simulink model "sampleModel7424"  (R2017a)
settings: Solver=VariableStepAuto  StartTime=0.0  StopTime=10.0  RelTol=1e-3
undefined symbols (not defined in the file): DiscIntNeverNeededParam
libraries: simulink x211
(part 1 of 4)
settings Model: Creator=cyfuzz  LastModifiedBy=cyfuzz

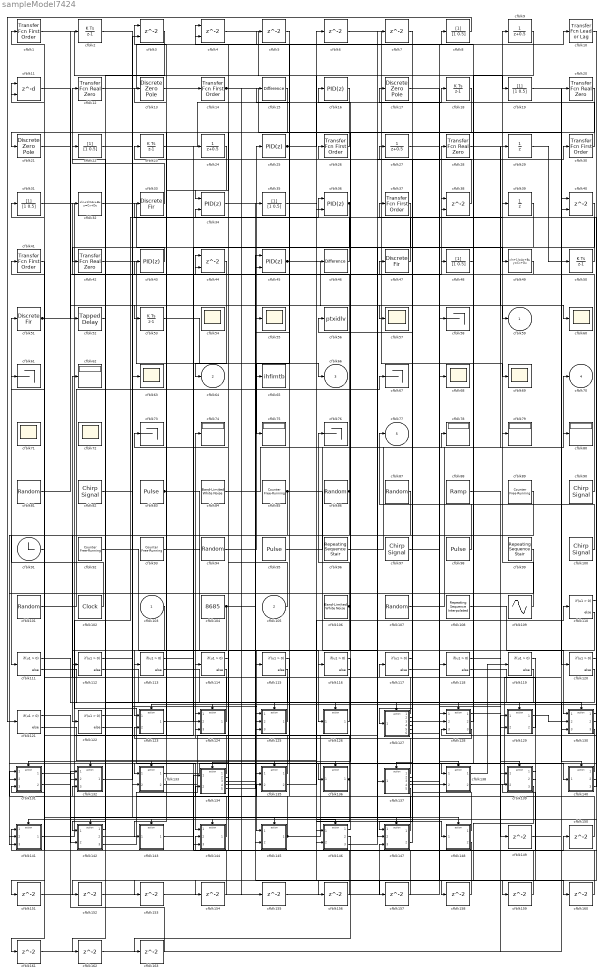
== system sampleModel7424 ==
  cfblk103 : Inport
  cfblk105 : Inport  Port=2
  cfblk{1,14,26,30,37,41} (6 alike) : simulink/Discrete/Transfer Fcn First Order  PoleZ=0.95  ICPrevOutput=0.0  DoSatur=off
      settings: SourceProductName=Simulink
  cfblk10 : simulink/Discrete/Transfer Fcn Lead or Lag  PoleZ=0.95  ZeroZ=0.75  ICPrevOutput=0.0  ICPrevInput=0.0  DoSatur=off
      settings: SourceProductName=Simulink  SourceProductBaseCode=SL
  cfblk{82,90,97,100} (4 alike) : simulink/Sources/Chirp Signal  f1=0.1  T=100  f2=1
  cfblk101 : UniformRandomNumber  SampleTime=0.1
  cfblk102 : DigitalClock
  cfblk104 : Constant  Value=8685
  cfblk106 : simulink/Sources/Band-Limited White Noise  Cov=[0.1]  Ts=0.1  seed=[23341]
  cfblk107 : RandomNumber  SampleTime=0.1
  cfblk108 : simulink/Sources/Repeating Sequence Interpolated  OutValues=[3 1 4 2 1].'  TimeValues=[0 0.1 0.5 0.6 1].'  LookUpMeth=Interpolation-Use End Values  tsamp=0.01  OutMin=[]  OutMax=[]  OutDataTypeStr=double  OutputDataTypeScalingMode=double  OutDataType=fixdt(0,8)  OutScaling=2^-10
  cfblk109 : Sin  SampleTime=0
  cfblk11 : Delay  DelayLengthSource=Input port  SampleTime=1
      settings: InputPortMap=u0,p1
  cfblk{110..122} (13 alike) : If  SampleTime=1
  cfblk{12,20,28,42} (4 alike) : simulink/Discrete/Transfer Fcn Real Zero  ZeroZ=0.75  ICPrevInput=0.0  DoSatur=off
      settings: SourceProductName=Simulink  SourceProductBaseCode=SL
  cfblk123 : Subsystem  TreatAsAtomicUnit=on
  cfblk124 : Subsystem  TreatAsAtomicUnit=on
  cfblk125 : Subsystem  TreatAsAtomicUnit=on
  cfblk126 : Subsystem  TreatAsAtomicUnit=on
  cfblk127 : Subsystem  TreatAsAtomicUnit=on
  cfblk128 : Subsystem  TreatAsAtomicUnit=on
  cfblk129 : Subsystem  TreatAsAtomicUnit=on
  cfblk13 : DiscreteZeroPole  Poles=[0 0.5]  Gain=1
  cfblk130 : Subsystem  TreatAsAtomicUnit=on
  cfblk131 : Subsystem  TreatAsAtomicUnit=on
  cfblk132 : Subsystem  TreatAsAtomicUnit=on
  cfblk133 : Subsystem  TreatAsAtomicUnit=on
  cfblk134 : Subsystem  TreatAsAtomicUnit=on
  cfblk135 : Subsystem  TreatAsAtomicUnit=on
  cfblk136 : Subsystem  TreatAsAtomicUnit=on
  cfblk137 : Subsystem  TreatAsAtomicUnit=on
  cfblk138 : Subsystem  TreatAsAtomicUnit=on
  cfblk139 : Subsystem  TreatAsAtomicUnit=on
  cfblk140 : Subsystem  TreatAsAtomicUnit=on
  cfblk141 : Subsystem  TreatAsAtomicUnit=on
  cfblk142 : Subsystem  TreatAsAtomicUnit=on
  cfblk143 : Subsystem  TreatAsAtomicUnit=on
  cfblk144 : Subsystem  TreatAsAtomicUnit=on
  cfblk145 : Subsystem  TreatAsAtomicUnit=on
  cfblk146 : Subsystem  TreatAsAtomicUnit=on
  cfblk147 : Subsystem  TreatAsAtomicUnit=on
  cfblk148 : Subsystem  TreatAsAtomicUnit=on
  cfblk{5..7,149..163} (18 alike) : Delay  SampleTime=1
  cfblk15 : simulink/Discrete/Difference  ICPrevInput=0.0  OutMin=[]  OutMax=[]  OutDataTypeStr=Inherit: Inherit via back propagation  OutDataType=fixdt(1, 16)  OutScaling=2^-10  DoSatur=off
  cfblk16 : simulink/Continuous/PID Controller  Controller=PID  TimeDomain=Discrete-time  SampleTime=1  IntegratorMethod=Forward Euler  FilterMethod=Forward Euler  Form=Parallel  UseFilter=on  ControllerParametersSource=internal  P=1  I=1  D=0  N=100  InitialConditionSource=internal  InitialConditionForIntegrator=0  InitialConditionForFilter=0  ExternalReset=none  LimitOutput=off  UpperSaturationLimit=inf  LowerSaturationLimit=-inf  LinearizeAsGain=off  AntiWindupMode=none  Kb=1  TrackingMode=off  Kt=1  PParamMin=[]  PParamMax=[]  IParamMin=[]  IParamMax=[]  DParamMin=[]  DParamMax=[]  NParamMin=[]  NParamMax=[]  KbParamMin=[]  KbParamMax=[]  KtParamMin=[]  KtParamMax=[]  POutMin=[]  POutMax=[]  IOutMin=[]  IOutMax=[]  DOutMin=[]  DOutMax=[]  NOutMin=[]  NOutMax=[]  KbOutMin=[]  KbOutMax=[]  KtOutMin=[]  KtOutMax=[]  IntegratorOutMin=[]  IntegratorOutMax=[]  FilterOutMin=[]  FilterOutMax=[]  SumOutMin=[]  SumOutMax=[]  SumI1OutMin=[]  SumI1OutMax=[]  SumI2OutMin=[]  SumI2OutMax=[]  SumI3OutMin=[]  SumI3OutMax=[]  SumDOutMin=[]  SumDOutMax=[]  SaturationOutMin=[]  SaturationOutMax=[]  IntegratorContinuousStateAttributes=''  IntegratorStateMustResolveToSignalObject=off  IntegratorRTWStateStorageClass=Auto  FilterContinuousStateAttributes=''  FilterStateMustResolveToSignalObject=off  FilterRTWStateStorageClass=Auto  DifferentiatorICPrevScaledInput=0  DifferentiatorOutMin=[]  DifferentiatorOutMax=[]  InitialConditionSetting=State (most efficient)
  cfblk17 : DiscreteZeroPole  Poles=[0 0.5]  Gain=1
  cfblk{2,18,23,50,53} (5 alike) : DiscreteIntegrator  InitialConditionSetting=State (most efficient)  ICPrevOutput=DiscIntNeverNeededParam  ICPrevScaledInput=DiscIntNeverNeededParam
  cfblk{8,19,22,31,35,48} (6 alike) : DiscreteFilter  SampleTime=1
  cfblk21 : DiscreteZeroPole  Poles=[0 0.5]  Gain=1
  cfblk24 : DiscreteTransferFcn  SampleTime=1
  cfblk25 : simulink/Continuous/PID Controller  Controller=PID  TimeDomain=Discrete-time  SampleTime=1  IntegratorMethod=Forward Euler  FilterMethod=Forward Euler  Form=Parallel  UseFilter=on  ControllerParametersSource=internal  P=1  I=1  D=0  N=100  InitialConditionSource=internal  InitialConditionForIntegrator=0  InitialConditionForFilter=0  ExternalReset=none  LimitOutput=off  UpperSaturationLimit=inf  LowerSaturationLimit=-inf  LinearizeAsGain=off  AntiWindupMode=none  Kb=1  TrackingMode=off  Kt=1  PParamMin=[]  PParamMax=[]  IParamMin=[]  IParamMax=[]  DParamMin=[]  DParamMax=[]  NParamMin=[]  NParamMax=[]  KbParamMin=[]  KbParamMax=[]  KtParamMin=[]  KtParamMax=[]  POutMin=[]  POutMax=[]  IOutMin=[]  IOutMax=[]  DOutMin=[]  DOutMax=[]  NOutMin=[]  NOutMax=[]  KbOutMin=[]  KbOutMax=[]  KtOutMin=[]  KtOutMax=[]  IntegratorOutMin=[]  IntegratorOutMax=[]  FilterOutMin=[]  FilterOutMax=[]  SumOutMin=[]  SumOutMax=[]  SumI1OutMin=[]  SumI1OutMax=[]  SumI2OutMin=[]  SumI2OutMax=[]  SumI3OutMin=[]  SumI3OutMax=[]  SumDOutMin=[]  SumDOutMax=[]  SaturationOutMin=[]  SaturationOutMax=[]  IntegratorContinuousStateAttributes=''  IntegratorStateMustResolveToSignalObject=off  IntegratorRTWStateStorageClass=Auto  FilterContinuousStateAttributes=''  FilterStateMustResolveToSignalObject=off  FilterRTWStateStorageClass=Auto  DifferentiatorICPrevScaledInput=0  DifferentiatorOutMin=[]  DifferentiatorOutMax=[]  InitialConditionSetting=State (most efficient)
  cfblk27 : DiscreteTransferFcn  SampleTime=1
  cfblk29 : UnitDelay
  cfblk{3..4,38,40,44} (5 alike) : Delay  ShowEnablePort=on  SampleTime=1
      settings: InputPortMap=u0,e6
  cfblk32 : DiscreteStateSpace
  cfblk33 : DiscreteFir  SampleTime=1
  cfblk34 : simulink/Continuous/PID Controller (2DOF)  Controller=PID  TimeDomain=Discrete-time  SampleTime=1  IntegratorMethod=Forward Euler  FilterMethod=Forward Euler  Form=Parallel  UseFilter=on  ControllerParametersSource=internal  P=1  I=1  D=0  N=100  b=1  c=1  InitialConditionSource=internal  InitialConditionForIntegrator=0  InitialConditionForFilter=0  ExternalReset=none  LimitOutput=off  UpperSaturationLimit=inf  LowerSaturationLimit=-inf  LinearizeAsGain=off  AntiWindupMode=none  Kb=1  TrackingMode=off  Kt=1  PParamMin=[]  PParamMax=[]  IParamMin=[]  IParamMax=[]  DParamMin=[]  DParamMax=[]  NParamMin=[]  NParamMax=[]  bParamMin=[]  bParamMax=[]  cParamMin=[]  cParamMax=[]  KbParamMin=[]  KbParamMax=[]  KtParamMin=[]  KtParamMax=[]  POutMin=[]  POutMax=[]  IOutMin=[]  IOutMax=[]  DOutMin=[]  DOutMax=[]  NOutMin=[]  NOutMax=[]  bOutMin=[]  bOutMax=[]  cOutMin=[]  cOutMax=[]  KbOutMin=[]  KbOutMax=[]  KtOutMin=[]  KtOutMax=[]  IntegratorOutMin=[]  IntegratorOutMax=[]  FilterOutMin=[]  FilterOutMax=[]  SumOutMin=[]  SumOutMax=[]  Sum1OutMin=[]  Sum1OutMax=[]  Sum2OutMin=[]  Sum2OutMax=[]  Sum3OutMin=[]  Sum3OutMax=[]  SumI1OutMin=[]  SumI1OutMax=[]  SumI2OutMin=[]  SumI2OutMax=[]  SumI3OutMin=[]  SumI3OutMax=[]  SumDOutMin=[]  SumDOutMax=[]  SaturationOutMin=[]  SaturationOutMax=[]  IntegratorContinuousStateAttributes=''  IntegratorStateMustResolveToSignalObject=off  IntegratorRTWStateStorageClass=Auto  FilterContinuousStateAttributes=''  FilterStateMustResolveToSignalObject=off  FilterRTWStateStorageClass=Auto  DifferentiatorICPrevScaledInput=0  DifferentiatorOutMin=[]  DifferentiatorOutMax=[]  InitialConditionSetting=State (most efficient)
  cfblk36 : simulink/Continuous/PID Controller (2DOF)  Controller=PID  TimeDomain=Discrete-time  SampleTime=1  IntegratorMethod=Forward Euler  FilterMethod=Forward Euler  Form=Parallel  UseFilter=on  ControllerParametersSource=internal  P=1  I=1  D=0  N=100  b=1  c=1  InitialConditionSource=internal  InitialConditionForIntegrator=0  InitialConditionForFilter=0  ExternalReset=none  LimitOutput=off  UpperSaturationLimit=inf  LowerSaturationLimit=-inf  LinearizeAsGain=off  AntiWindupMode=none  Kb=1  TrackingMode=off  Kt=1  PParamMin=[]  PParamMax=[]  IParamMin=[]  IParamMax=[]  DParamMin=[]  DParamMax=[]  NParamMin=[]  NParamMax=[]  bParamMin=[]  bParamMax=[]  cParamMin=[]  cParamMax=[]  KbParamMin=[]  KbParamMax=[]  KtParamMin=[]  KtParamMax=[]  POutMin=[]  POutMax=[]  IOutMin=[]  IOutMax=[]  DOutMin=[]  DOutMax=[]  NOutMin=[]  NOutMax=[]  bOutMin=[]  bOutMax=[]  cOutMin=[]  cOutMax=[]  KbOutMin=[]  KbOutMax=[]  KtOutMin=[]  KtOutMax=[]  IntegratorOutMin=[]  IntegratorOutMax=[]  FilterOutMin=[]  FilterOutMax=[]  SumOutMin=[]  SumOutMax=[]  Sum1OutMin=[]  Sum1OutMax=[]  Sum2OutMin=[]  Sum2OutMax=[]  Sum3OutMin=[]  Sum3OutMax=[]  SumI1OutMin=[]  SumI1OutMax=[]  SumI2OutMin=[]  SumI2OutMax=[]  SumI3OutMin=[]  SumI3OutMax=[]  SumDOutMin=[]  SumDOutMax=[]  SaturationOutMin=[]  SaturationOutMax=[]  IntegratorContinuousStateAttributes=''  IntegratorStateMustResolveToSignalObject=off  IntegratorRTWStateStorageClass=Auto  FilterContinuousStateAttributes=''  FilterStateMustResolveToSignalObject=off  FilterRTWStateStorageClass=Auto  DifferentiatorICPrevScaledInput=0  DifferentiatorOutMin=[]  DifferentiatorOutMax=[]  InitialConditionSetting=State (most efficient)
  cfblk39 : UnitDelay
  cfblk43 : simulink/Continuous/PID Controller  Controller=PID  TimeDomain=Discrete-time  SampleTime=1  IntegratorMethod=Forward Euler  FilterMethod=Forward Euler  Form=Parallel  UseFilter=on  ControllerParametersSource=internal  P=1  I=1  D=0  N=100  InitialConditionSource=internal  InitialConditionForIntegrator=0  InitialConditionForFilter=0  ExternalReset=none  LimitOutput=off  UpperSaturationLimit=inf  LowerSaturationLimit=-inf  LinearizeAsGain=off  AntiWindupMode=none  Kb=1  TrackingMode=off  Kt=1  PParamMin=[]  PParamMax=[]  IParamMin=[]  IParamMax=[]  DParamMin=[]  DParamMax=[]  NParamMin=[]  NParamMax=[]  KbParamMin=[]  KbParamMax=[]  KtParamMin=[]  KtParamMax=[]  POutMin=[]  POutMax=[]  IOutMin=[]  IOutMax=[]  DOutMin=[]  DOutMax=[]  NOutMin=[]  NOutMax=[]  KbOutMin=[]  KbOutMax=[]  KtOutMin=[]  KtOutMax=[]  IntegratorOutMin=[]  IntegratorOutMax=[]  FilterOutMin=[]  FilterOutMax=[]  SumOutMin=[]  SumOutMax=[]  SumI1OutMin=[]  SumI1OutMax=[]  SumI2OutMin=[]  SumI2OutMax=[]  SumI3OutMin=[]  SumI3OutMax=[]  SumDOutMin=[]  SumDOutMax=[]  SaturationOutMin=[]  SaturationOutMax=[]  IntegratorContinuousStateAttributes=''  IntegratorStateMustResolveToSignalObject=off  IntegratorRTWStateStorageClass=Auto  FilterContinuousStateAttributes=''  FilterStateMustResolveToSignalObject=off  FilterRTWStateStorageClass=Auto  DifferentiatorICPrevScaledInput=0  DifferentiatorOutMin=[]  DifferentiatorOutMax=[]  InitialConditionSetting=State (most efficient)
  cfblk45 : simulink/Continuous/PID Controller (2DOF)  Controller=PID  TimeDomain=Discrete-time  SampleTime=1  IntegratorMethod=Forward Euler  FilterMethod=Forward Euler  Form=Parallel  UseFilter=on  ControllerParametersSource=internal  P=1  I=1  D=0  N=100  b=1  c=1  InitialConditionSource=internal  InitialConditionForIntegrator=0  InitialConditionForFilter=0  ExternalReset=none  LimitOutput=off  UpperSaturationLimit=inf  LowerSaturationLimit=-inf  LinearizeAsGain=off  AntiWindupMode=none  Kb=1  TrackingMode=off  Kt=1  PParamMin=[]  PParamMax=[]  IParamMin=[]  IParamMax=[]  DParamMin=[]  DParamMax=[]  NParamMin=[]  NParamMax=[]  bParamMin=[]  bParamMax=[]  cParamMin=[]  cParamMax=[]  KbParamMin=[]  KbParamMax=[]  KtParamMin=[]  KtParamMax=[]  POutMin=[]  POutMax=[]  IOutMin=[]  IOutMax=[]  DOutMin=[]  DOutMax=[]  NOutMin=[]  NOutMax=[]  bOutMin=[]  bOutMax=[]  cOutMin=[]  cOutMax=[]  KbOutMin=[]  KbOutMax=[]  KtOutMin=[]  KtOutMax=[]  IntegratorOutMin=[]  IntegratorOutMax=[]  FilterOutMin=[]  FilterOutMax=[]  SumOutMin=[]  SumOutMax=[]  Sum1OutMin=[]  Sum1OutMax=[]  Sum2OutMin=[]  Sum2OutMax=[]  Sum3OutMin=[]  Sum3OutMax=[]  SumI1OutMin=[]  SumI1OutMax=[]  SumI2OutMin=[]  SumI2OutMax=[]  SumI3OutMin=[]  SumI3OutMax=[]  SumDOutMin=[]  SumDOutMax=[]  SaturationOutMin=[]  SaturationOutMax=[]  IntegratorContinuousStateAttributes=''  IntegratorStateMustResolveToSignalObject=off  IntegratorRTWStateStorageClass=Auto  FilterContinuousStateAttributes=''  FilterStateMustResolveToSignalObject=off  FilterRTWStateStorageClass=Auto  DifferentiatorICPrevScaledInput=0  DifferentiatorOutMin=[]  DifferentiatorOutMax=[]  InitialConditionSetting=State (most efficient)
  cfblk46 : simulink/Discrete/Difference  ICPrevInput=0.0  OutMin=[]  OutMax=[]  OutDataTypeStr=Inherit: Inherit via back propagation  OutDataType=fixdt(1, 16)  OutScaling=2^-10  DoSatur=off
  cfblk47 : DiscreteFir  SampleTime=1
  cfblk49 : DiscreteStateSpace
  cfblk51 : DiscreteFir  SampleTime=1
  cfblk52 : simulink/Discrete/Tapped Delay  vinit=0.0  samptime=-1  NumDelays=1  DelayOrder=Oldest  includeCurrent=off
  cfblk{54..55,57,60,63,68..69,71..72} (9 alike) : Scope
      cfblk54 settings: Floating=on
      cfblk71 settings: Floating=on
      cfblk72 settings: Floating=on
  cfblk56 : ToWorkspace  VariableName=ptxidlv  SaveFormat=Timeseries  SampleTime=-1
  cfblk{58,61,67,73,76} (5 alike) : Terminator
  cfblk{62,74..75,78..80} (6 alike) : Display
  cfblk65 : ToWorkspace  VariableName=ihfimtb  SaveFormat=Timeseries  SampleTime=-1
  cfblk81 : RandomNumber  SampleTime=0.1
  cfblk83 : DiscretePulseGenerator  PulseType=Time based  Period=10  PulseWidth=5
  cfblk84 : simulink/Sources/Band-Limited White Noise  Cov=[0.1]  Ts=0.1  seed=[23341]
  cfblk{85,89,92..93} (4 alike) : simulink/Sources/Counter Free-Running  NumBits=16  tsamp=-1
  cfblk86 : UniformRandomNumber  SampleTime=0.1
  cfblk87 : RandomNumber  SampleTime=0.1
  cfblk88 : simulink/Sources/Ramp  slope=1  start=0  X0=0
  cfblk9 : DiscreteTransferFcn  SampleTime=1
  cfblk91 : Clock
  cfblk94 : UniformRandomNumber  SampleTime=0.1
  cfblk95 : DiscretePulseGenerator  PulseType=Time based  Period=10  PulseWidth=5
  cfblk96 : simulink/Sources/Repeating Sequence Stair  OutValues=[3 1 4 2 1].'  tsamp=-1  OutMin=[]  OutMax=[]  OutDataTypeStr=double  OutputDataTypeScalingMode=double  OutDataType=fixdt(0,8)  ConRadixGroup=Best Precision: Vector-wise  OutScaling=2^-12
  cfblk98 : DiscretePulseGenerator  PulseType=Time based  Period=10  PulseWidth=5
  cfblk99 : simulink/Sources/Repeating Sequence Stair  OutValues=[3 1 4 2 1].'  tsamp=-1  OutMin=[]  OutMax=[]  OutDataTypeStr=double  OutputDataTypeScalingMode=double  OutDataType=fixdt(0,8)  ConRadixGroup=Best Precision: Vector-wise  OutScaling=2^-12
  cfblk59 : Outport
  cfblk64 : Outport  Port=2
  cfblk66 : Outport  Port=3
  cfblk70 : Outport  Port=4
  cfblk77 : Outport  Port=5
  wires:
  cfblk29/1 -> cfblk50/1
  cfblk23/1 -> cfblk18/1
  cfblk48/1 -> cfblk4/1
  cfblk109/1 -> cfblk9/1
  cfblk93/1 -> cfblk126/1(cfblk1)
  cfblk100/1 -> cfblk77/1
  cfblk138/1(cfblk2) -> cfblk119/1
  cfblk105/1 -> cfblk73/1
  cfblk102/1 -> cfblk51/1
  cfblk141/1(cfblk2) -> cfblk36/1
  cfblk92/1 -> cfblk145/1(cfblk1)
  cfblk42/1 -> cfblk66/1
  cfblk50/1 -> cfblk16/1
  cfblk83/1 -> cfblk115/1, cfblk146/1(cfblk1)
  cfblk94/1 -> cfblk25/1
  cfblk87/1 -> cfblk111/1
  cfblk84/1 -> cfblk78/1
  cfblk8/1 -> cfblk121/1
  cfblk45/1 -> cfblk59/1, cfblk5/1
  cfblk126/1(cfblk2) -> cfblk23/1
  cfblk33/1 -> cfblk12/1
  cfblk12/1 -> cfblk8/1
  cfblk95/1 -> cfblk70/1
  cfblk6/1 -> cfblk69/1
  cfblk108/1 -> cfblk130/1(cfblk1)
  cfblk146/1(cfblk2) -> cfblk26/1
  cfblk25/1 -> cfblk6/1, cfblk148/1(cfblk1)
  cfblk132/1(cfblk2) -> cfblk63/1
  cfblk4/1 -> cfblk19/1
  cfblk20/1 -> cfblk116/1
  cfblk14/1 -> cfblk120/1, cfblk155/1
  cfblk96/1 -> cfblk29/1
  cfblk13/1 -> cfblk14/1
  cfblk10/1 -> cfblk141/1(cfblk1)
  cfblk15/1 -> cfblk133/1(cfblk1)
  cfblk17/1 -> cfblk58/1
  cfblk53/1 -> cfblk75/1
  cfblk89/1 -> cfblk122/1
  cfblk98/1 -> cfblk47/1
  cfblk7/1 -> cfblk127/1(cfblk1)
  cfblk31/1 -> cfblk144/1(cfblk1)
  cfblk136/1(cfblk2) -> cfblk1/1, cfblk146/2(cfblk10)
  cfblk47/1 -> cfblk37/1
  cfblk124/1(cfblk2) -> cfblk61/1
  cfblk138/2(cfblk7) -> cfblk20/1
  cfblk137/1(cfblk2) -> cfblk55/1
  cfblk134/1(cfblk2) -> cfblk43/1
  cfblk9/1 -> cfblk138/1(cfblk1)
  cfblk30/1 -> cfblk17/1
  cfblk133/1(cfblk2) -> cfblk140/1(cfblk1)
  cfblk123/1(cfblk2) -> cfblk74/1
  cfblk38/1 -> cfblk13/1
  cfblk101/1 -> cfblk7/1
  cfblk97/1 -> cfblk138/2(cfblk6)
  cfblk5/1 -> cfblk65/1
  cfblk46/1 -> cfblk3/1
  cfblk3/1 -> cfblk142/1(cfblk1)
  cfblk1/1 -> cfblk46/1
  cfblk44/1 -> cfblk64/1
  cfblk16/1 -> cfblk36/2
  cfblk91/1 -> cfblk31/1
  cfblk145/1(cfblk2) -> cfblk79/1, cfblk132/3(cfblk14)
  cfblk131/1(cfblk2) -> cfblk24/1
  cfblk81/1 -> cfblk2/1
  cfblk144/1(cfblk2) -> cfblk41/1
  cfblk86/1 -> cfblk32/1, cfblk141/3(cfblk14)
  cfblk21/1 -> cfblk52/1
  cfblk148/1(cfblk2) -> cfblk27/1
  cfblk51/1 -> cfblk11/1, cfblk48/1
  cfblk82/1 -> cfblk3/2
  cfblk137/2(cfblk11) -> cfblk35/1
  cfblk127/1(cfblk2) -> cfblk11/2
  cfblk90/1 -> cfblk28/1
  cfblk103/1 -> cfblk123/1(cfblk1)
  cfblk18/1 -> cfblk34/1
  cfblk2/1 -> cfblk57/1
  cfblk28/1 -> cfblk60/1
  cfblk127/2(cfblk13) -> cfblk123/2(cfblk10)
  cfblk106/1 -> cfblk76/1, cfblk125/2(cfblk9)
  cfblk129/1(cfblk2) -> cfblk130/2(cfblk7)
  cfblk43/1 -> cfblk42/1
  cfblk148/2(cfblk17) -> cfblk144/2(cfblk12)
  cfblk11/1 -> cfblk53/1
  cfblk135/1(cfblk2) -> cfblk124/1(cfblk1)
  cfblk134/2(cfblk14) -> cfblk34/2
  cfblk127/3(cfblk14) -> cfblk10/1
  cfblk134/3(cfblk15) -> cfblk45/1
  cfblk19/1 -> cfblk40/2
  cfblk142/1(cfblk2) -> cfblk22/1
  cfblk131/2(cfblk15) -> cfblk142/2(cfblk13)
  cfblk129/2(cfblk9) -> cfblk117/1
  cfblk107/1 -> cfblk80/1
  cfblk39/1 -> cfblk145/2(cfblk16)
  cfblk26/1 -> cfblk21/1
  cfblk32/1 -> cfblk49/1
  cfblk147/1(cfblk2) -> cfblk15/1
  cfblk128/2(cfblk11) -> cfblk38/1
  cfblk104/1 -> cfblk135/1(cfblk1), cfblk112/1
  cfblk27/1 -> cfblk129/2(cfblk8)
  cfblk36/1 -> cfblk124/2(cfblk12), cfblk125/3(cfblk10)
  cfblk85/1 -> cfblk137/1(cfblk1), cfblk143/1(cfblk1), cfblk133/2(cfblk16)
  cfblk40/1 -> cfblk147/1(cfblk1)
  cfblk134/4(cfblk16) -> cfblk67/1
  cfblk147/2(cfblk12) -> cfblk44/1
  cfblk142/2(cfblk14) -> cfblk39/1
  cfblk125/1(cfblk2) -> cfblk62/1
  cfblk99/1 -> cfblk141/2(cfblk13)
  cfblk49/1 -> cfblk44/2
  cfblk22/1 -> cfblk125/1(cfblk1)
  cfblk37/1 -> cfblk147/2(cfblk10)
  cfblk146/3(cfblk12) -> cfblk30/1
  cfblk133/2(cfblk17) -> cfblk38/2
  cfblk128/3(cfblk12) -> cfblk124/3(cfblk13)
  cfblk127/4(cfblk15) -> cfblk56/1
  cfblk127/5(cfblk16) -> cfblk136/1(cfblk1)
  cfblk88/1 -> cfblk139/1(cfblk1)
  cfblk142/3(cfblk15) -> cfblk135/2(cfblk13)
  cfblk140/1(cfblk2) -> cfblk131/2(cfblk13)
  cfblk140/2(cfblk7) -> cfblk132/2(cfblk13)
  cfblk130/1(cfblk2) -> cfblk128/3(cfblk10)
  cfblk140/3(cfblk8) -> cfblk33/1
  cfblk127/6(cfblk17) -> cfblk68/1
  cfblk135/2(cfblk14) -> cfblk110/1
  cfblk134/5(cfblk17) -> cfblk45/2
  cfblk24/1 -> cfblk113/1
  cfblk130/3(cfblk10) -> cfblk144/3(cfblk13)
  cfblk110/1 -> cfblk123/Action
  cfblk110/2 -> cfblk124/Action
  cfblk111/1 -> cfblk125/Action
  cfblk111/2 -> cfblk126/Action
  cfblk112/1 -> cfblk127/Action
  cfblk112/2 -> cfblk128/Action
  cfblk113/1 -> cfblk129/Action
  cfblk113/2 -> cfblk130/Action
  cfblk114/1 -> cfblk131/Action
  cfblk114/2 -> cfblk132/Action
  cfblk115/1 -> cfblk133/Action
  cfblk115/2 -> cfblk134/Action
  cfblk116/1 -> cfblk135/Action
  cfblk116/2 -> cfblk136/Action
  cfblk117/1 -> cfblk137/Action
  cfblk117/2 -> cfblk138/Action
  cfblk118/1 -> cfblk139/Action
  cfblk118/2 -> cfblk140/Action
  cfblk119/1 -> cfblk141/Action
  cfblk119/2 -> cfblk142/Action
  cfblk120/1 -> cfblk143/Action
  cfblk120/2 -> cfblk144/Action
  cfblk121/1 -> cfblk145/Action
  cfblk121/2 -> cfblk146/Action
  cfblk122/1 -> cfblk147/Action
  cfblk122/2 -> cfblk148/Action
  cfblk128/1(cfblk2) -> cfblk149/1
  cfblk149/1 -> cfblk40/1
  cfblk143/1(cfblk2) -> cfblk150/1
  cfblk150/1 -> cfblk131/1(cfblk1)
  cfblk41/1 -> cfblk151/1
  cfblk151/1 -> cfblk128/2(cfblk9)
  cfblk139/1(cfblk2) -> cfblk152/1
  cfblk152/1 -> cfblk128/1(cfblk1)
  cfblk139/2(cfblk9) -> cfblk153/1
  cfblk153/1 -> cfblk147/3(cfblk11)
  cfblk139/3(cfblk10) -> cfblk154/1
  cfblk154/1 -> cfblk131/3(cfblk14)
  cfblk155/1 -> cfblk118/1
  cfblk130/2(cfblk9) -> cfblk156/1
  cfblk156/1 -> cfblk134/2(cfblk13)
  cfblk34/1 -> cfblk157/1
  cfblk157/1 -> cfblk114/1
  cfblk35/1 -> cfblk158/1
  cfblk158/1 -> cfblk4/2
  cfblk137/3(cfblk12) -> cfblk159/1
  cfblk159/1 -> cfblk134/1(cfblk1)
  cfblk137/4(cfblk13) -> cfblk160/1
  cfblk160/1 -> cfblk139/2(cfblk8)
  cfblk137/5(cfblk14) -> cfblk161/1
  cfblk161/1 -> cfblk130/3(cfblk8)
  cfblk52/1 -> cfblk162/1
  cfblk162/1 -> cfblk129/1(cfblk1)
  cfblk146/2(cfblk11) -> cfblk163/1
  cfblk163/1 -> cfblk132/1(cfblk1)

== system sampleModel7424/cfblk123 ==
  cfblk1 : Inport
  cfblk10 : Inport  Port=2
  Action Port : ActionPort  ActionType=then
  cfblk3 : UnitDelay  SampleTime=-1
  cfblk4 : simulink/Continuous/PID Controller  Controller=PID  TimeDomain=Discrete-time  SampleTime=-1  IntegratorMethod=Forward Euler  FilterMethod=Forward Euler  Form=Parallel  UseFilter=on  ControllerParametersSource=internal  P=1  I=1  D=0  N=100  InitialConditionSource=internal  InitialConditionForIntegrator=0  InitialConditionForFilter=0  ExternalReset=none  LimitOutput=off  UpperSaturationLimit=inf  LowerSaturationLimit=-inf  LinearizeAsGain=off  AntiWindupMode=none  Kb=1  TrackingMode=off  Kt=1  PParamMin=[]  PParamMax=[]  IParamMin=[]  IParamMax=[]  DParamMin=[]  DParamMax=[]  NParamMin=[]  NParamMax=[]  KbParamMin=[]  KbParamMax=[]  KtParamMin=[]  KtParamMax=[]  POutMin=[]  POutMax=[]  IOutMin=[]  IOutMax=[]  DOutMin=[]  DOutMax=[]  NOutMin=[]  NOutMax=[]  KbOutMin=[]  KbOutMax=[]  KtOutMin=[]  KtOutMax=[]  IntegratorOutMin=[]  IntegratorOutMax=[]  FilterOutMin=[]  FilterOutMax=[]  SumOutMin=[]  SumOutMax=[]  SumI1OutMin=[]  SumI1OutMax=[]  SumI2OutMin=[]  SumI2OutMax=[]  SumI3OutMin=[]  SumI3OutMax=[]  SumDOutMin=[]  SumDOutMax=[]  SaturationOutMin=[]  SaturationOutMax=[]  IntegratorContinuousStateAttributes=''  IntegratorStateMustResolveToSignalObject=off  IntegratorRTWStateStorageClass=Auto  FilterContinuousStateAttributes=''  FilterStateMustResolveToSignalObject=off  FilterRTWStateStorageClass=Auto  DifferentiatorICPrevScaledInput=0  DifferentiatorOutMin=[]  DifferentiatorOutMax=[]  InitialConditionSetting=State (most efficient)
  cfblk5 : DiscreteTransferFcn
  cfblk6 : DiscreteIntegrator  InitialConditionSetting=State (most efficient)  SampleTime=-1  ICPrevOutput=DiscIntNeverNeededParam  ICPrevScaledInput=DiscIntNeverNeededParam
  cfblk7 : Delay
  cfblk8 : simulink/Discrete/Tapped Delay  vinit=0.0  samptime=-1  NumDelays=1  DelayOrder=Oldest  includeCurrent=off
  cfblk9 : DiscreteTransferFcn
  cfblk2 : Outport
  wires:
  cfblk4/1 -> cfblk8/1
  cfblk9/1 -> cfblk2/1
  cfblk6/1 -> cfblk7/1
  cfblk7/1 -> cfblk3/1
  cfblk10/1 -> cfblk4/1
  cfblk1/1 -> cfblk9/1
  cfblk3/1 -> cfblk5/1
  cfblk8/1 -> cfblk6/1

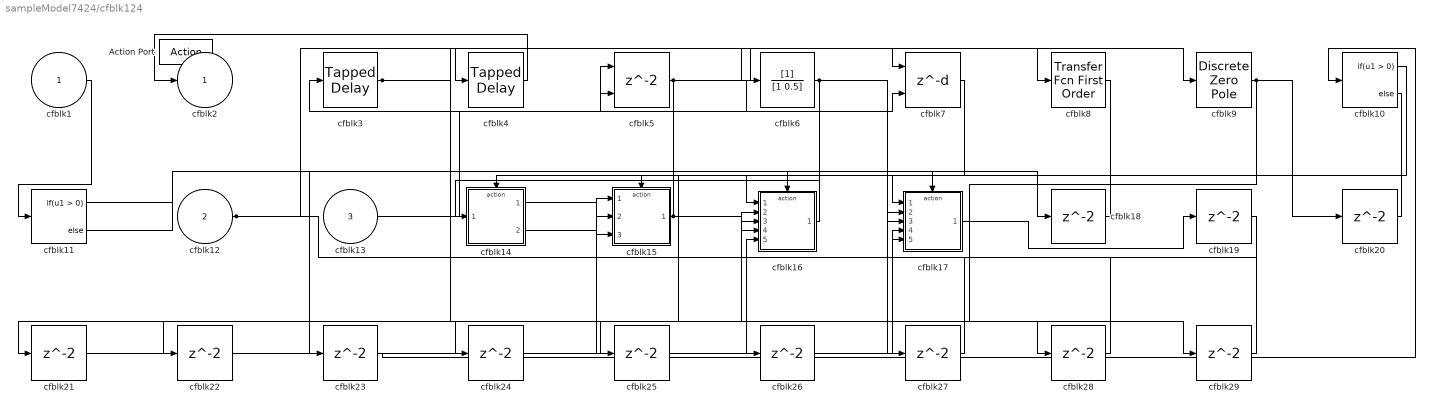
== system sampleModel7424/cfblk124 ==
  cfblk1 : Inport
  cfblk12 : Inport  Port=2
  cfblk13 : Inport  Port=3
  Action Port : ActionPort  ActionType=else
  cfblk10 : If  SampleTime=1
  cfblk11 : If  SampleTime=1
  cfblk14 : Subsystem  TreatAsAtomicUnit=on
  cfblk15 : Subsystem  TreatAsAtomicUnit=on
  cfblk16 : Subsystem  TreatAsAtomicUnit=on
  cfblk17 : Subsystem  TreatAsAtomicUnit=on
  cfblk{18..29} (12 alike) : Delay
  cfblk3 : simulink/Discrete/Tapped Delay  vinit=0.0  samptime=-1  NumDelays=1  DelayOrder=Oldest  includeCurrent=off
  cfblk4 : simulink/Discrete/Tapped Delay  vinit=0.0  samptime=-1  NumDelays=1  DelayOrder=Oldest  includeCurrent=off
  cfblk5 : Delay  ShowEnablePort=on
      settings: InputPortMap=u0,e6
  cfblk6 : DiscreteFilter
  cfblk7 : Delay  DelayLengthSource=Input port
      settings: InputPortMap=u0,p1
  cfblk8 : simulink/Discrete/Transfer Fcn First Order  PoleZ=0.95  ICPrevOutput=0.0  DoSatur=off
      settings: SourceProductName=Simulink
  cfblk9 : DiscreteZeroPole  Poles=[0 0.5]  Gain=1  SampleTime=-1
  cfblk2 : Outport
  wires:
  cfblk15/1(cfblk2) -> cfblk3/1, cfblk5/1, cfblk27/1
  cfblk1/1 -> cfblk11/1
  cfblk5/1 -> cfblk7/1, cfblk8/1, cfblk23/1
  cfblk12/1 -> cfblk4/1, cfblk17/4(cfblk14)
  cfblk13/1 -> cfblk7/2
  cfblk16/1(cfblk2) -> cfblk6/1
  cfblk3/1 -> cfblk9/1, cfblk5/2, cfblk18/1, cfblk25/1, cfblk26/1
  cfblk14/1(cfblk2) -> cfblk15/3(cfblk16)
  cfblk9/1 -> cfblk20/1, cfblk21/1
  cfblk6/1 -> cfblk14/1(cfblk1), cfblk29/1
  cfblk4/1 -> cfblk2/1
  cfblk10/1 -> cfblk14/Action
  cfblk10/2 -> cfblk15/Action
  cfblk11/1 -> cfblk16/Action
  cfblk11/2 -> cfblk17/Action
  cfblk18/1 -> cfblk17/1(cfblk1)
  cfblk17/1(cfblk2) -> cfblk19/1
  cfblk19/1 -> cfblk15/2(cfblk15)
  cfblk20/1 -> cfblk16/1(cfblk1)
  cfblk21/1 -> cfblk17/3(cfblk13)
  cfblk7/1 -> cfblk22/1
  cfblk22/1 -> cfblk17/2(cfblk12)
  cfblk23/1 -> cfblk10/1
  cfblk8/1 -> cfblk24/1
  cfblk24/1 -> cfblk15/1(cfblk1)
  cfblk25/1 -> cfblk16/5(cfblk14)
  cfblk26/1 -> cfblk17/5(cfblk15)
  cfblk27/1 -> cfblk16/3(cfblk12)
  cfblk14/2(cfblk7) -> cfblk28/1
  cfblk28/1 -> cfblk16/2(cfblk11)
  cfblk29/1 -> cfblk16/4(cfblk13)

== system sampleModel7424/cfblk125 ==
  cfblk1 : Inport
  cfblk9 : Inport  Port=2
  cfblk10 : Inport  Port=3
  Action Port : ActionPort  ActionType=then
  cfblk11 : Subsystem  TreatAsAtomicUnit=on
  cfblk12 : Subsystem  TreatAsAtomicUnit=on
  cfblk13 : Delay
  cfblk14 : Delay
  cfblk3 : simulink/Discrete/Transfer Fcn Real Zero  ZeroZ=0.75  ICPrevInput=0.0  DoSatur=off
      settings: SourceProductName=Simulink  SourceProductBaseCode=SL
  cfblk4 : Delay  DelayLengthSource=Input port
      settings: InputPortMap=u0,p1
  cfblk5 : simulink/Discrete/Transfer Fcn Lead or Lag  PoleZ=0.95  ZeroZ=0.75  ICPrevOutput=0.0  ICPrevInput=0.0  DoSatur=off
      settings: SourceProductName=Simulink  SourceProductBaseCode=SL
  cfblk6 : simulink/Discrete/Transfer Fcn Lead or Lag  PoleZ=0.95  ZeroZ=0.75  ICPrevOutput=0.0  ICPrevInput=0.0  DoSatur=off
      settings: SourceProductName=Simulink  SourceProductBaseCode=SL
  cfblk7 : DiscreteIntegrator  InitialConditionSetting=State (most efficient)  SampleTime=-1  ICPrevOutput=DiscIntNeverNeededParam  ICPrevScaledInput=DiscIntNeverNeededParam
  cfblk8 : If  SampleTime=1
  cfblk2 : Outport
  wires:
  cfblk4/1 -> cfblk5/1
  cfblk7/1 -> cfblk12/1(cfblk1)
  cfblk9/1 -> cfblk6/1
  cfblk10/1 -> cfblk2/1
  cfblk6/1 -> cfblk3/1
  cfblk11/2(cfblk13) -> cfblk4/2
  cfblk1/1 -> cfblk7/1
  cfblk3/1 -> cfblk11/1(cfblk1)
  cfblk12/1(cfblk2) -> cfblk11/2(cfblk12)
  cfblk8/1 -> cfblk11/Action
  cfblk8/2 -> cfblk12/Action
  cfblk11/1(cfblk2) -> cfblk13/1
  cfblk13/1 -> cfblk8/1
  cfblk5/1 -> cfblk14/1
  cfblk14/1 -> cfblk4/1

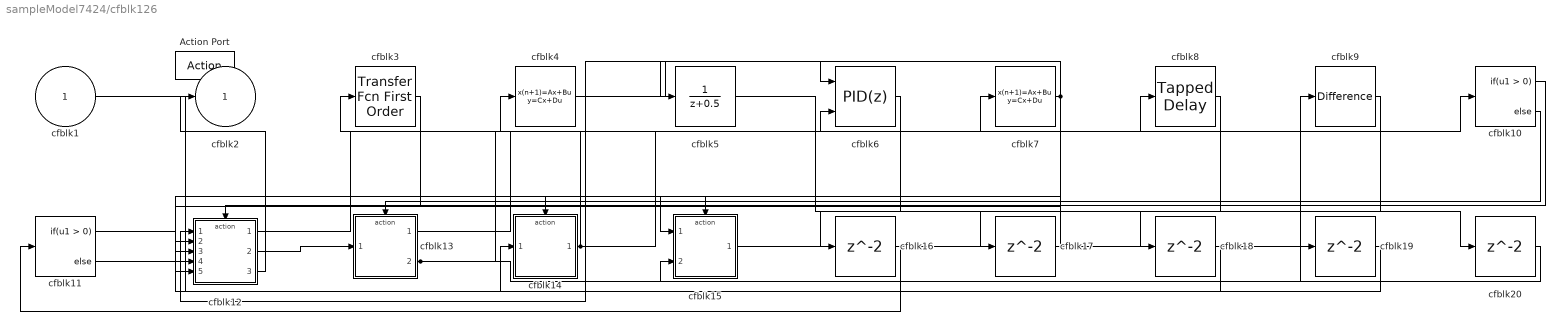
== system sampleModel7424/cfblk126 ==
  cfblk1 : Inport
  Action Port : ActionPort  ActionType=else
  cfblk10 : If  SampleTime=1
  cfblk11 : If  SampleTime=1
  cfblk12 : Subsystem  TreatAsAtomicUnit=on
  cfblk13 : Subsystem  TreatAsAtomicUnit=on
  cfblk14 : Subsystem  TreatAsAtomicUnit=on
  cfblk15 : Subsystem  TreatAsAtomicUnit=on
  cfblk{16..20} (5 alike) : Delay
  cfblk3 : simulink/Discrete/Transfer Fcn First Order  PoleZ=0.95  ICPrevOutput=0.0  DoSatur=off
      settings: SourceProductName=Simulink
  cfblk4 : DiscreteStateSpace  SampleTime=-1
  cfblk5 : DiscreteTransferFcn
  cfblk6 : simulink/Continuous/PID Controller (2DOF)  Controller=PID  TimeDomain=Discrete-time  SampleTime=-1  IntegratorMethod=Forward Euler  FilterMethod=Forward Euler  Form=Parallel  UseFilter=on  ControllerParametersSource=internal  P=1  I=1  D=0  N=100  b=1  c=1  InitialConditionSource=internal  InitialConditionForIntegrator=0  InitialConditionForFilter=0  ExternalReset=none  LimitOutput=off  UpperSaturationLimit=inf  LowerSaturationLimit=-inf  LinearizeAsGain=off  AntiWindupMode=none  Kb=1  TrackingMode=off  Kt=1  PParamMin=[]  PParamMax=[]  IParamMin=[]  IParamMax=[]  DParamMin=[]  DParamMax=[]  NParamMin=[]  NParamMax=[]  bParamMin=[]  bParamMax=[]  cParamMin=[]  cParamMax=[]  KbParamMin=[]  KbParamMax=[]  KtParamMin=[]  KtParamMax=[]  POutMin=[]  POutMax=[]  IOutMin=[]  IOutMax=[]  DOutMin=[]  DOutMax=[]  NOutMin=[]  NOutMax=[]  bOutMin=[]  bOutMax=[]  cOutMin=[]  cOutMax=[]  KbOutMin=[]  KbOutMax=[]  KtOutMin=[]  KtOutMax=[]  IntegratorOutMin=[]  IntegratorOutMax=[]  FilterOutMin=[]  FilterOutMax=[]  SumOutMin=[]  SumOutMax=[]  Sum1OutMin=[]  Sum1OutMax=[]  Sum2OutMin=[]  Sum2OutMax=[]  Sum3OutMin=[]  Sum3OutMax=[]  SumI1OutMin=[]  SumI1OutMax=[]  SumI2OutMin=[]  SumI2OutMax=[]  SumI3OutMin=[]  SumI3OutMax=[]  SumDOutMin=[]  SumDOutMax=[]  SaturationOutMin=[]  SaturationOutMax=[]  IntegratorContinuousStateAttributes=''  IntegratorStateMustResolveToSignalObject=off  IntegratorRTWStateStorageClass=Auto  FilterContinuousStateAttributes=''  FilterStateMustResolveToSignalObject=off  FilterRTWStateStorageClass=Auto  DifferentiatorICPrevScaledInput=0  DifferentiatorOutMin=[]  DifferentiatorOutMax=[]  InitialConditionSetting=State (most efficient)
  cfblk7 : DiscreteStateSpace  SampleTime=-1
  cfblk8 : simulink/Discrete/Tapped Delay  vinit=0.0  samptime=-1  NumDelays=1  DelayOrder=Oldest  includeCurrent=off
  cfblk9 : simulink/Discrete/Difference  ICPrevInput=0.0  OutMin=[]  OutMax=[]  OutDataTypeStr=Inherit: Inherit via back propagation  OutDataType=fixdt(1, 16)  OutScaling=2^-10  DoSatur=off
  cfblk2 : Outport
  wires:
  cfblk12/1(cfblk2) -> cfblk4/1
  cfblk1/1 -> cfblk14/1(cfblk1)
  cfblk7/1 -> cfblk12/1(cfblk1), cfblk5/1, cfblk12/5(cfblk13)
  cfblk12/2(cfblk14) -> cfblk13/1(cfblk1)
  cfblk4/1 -> cfblk6/1
  cfblk13/1(cfblk2) -> cfblk8/1
  cfblk14/1(cfblk2) -> cfblk10/1, cfblk3/1, cfblk7/1
  cfblk15/1(cfblk2) -> cfblk9/1
  cfblk3/1 -> cfblk12/2(cfblk10)
  cfblk13/2(cfblk7) -> cfblk6/2, cfblk19/1
  cfblk12/3(cfblk15) -> cfblk2/1
  cfblk10/1 -> cfblk12/Action
  cfblk10/2 -> cfblk13/Action
  cfblk11/1 -> cfblk14/Action
  cfblk11/2 -> cfblk15/Action
  cfblk6/1 -> cfblk16/1
  cfblk16/1 -> cfblk11/1
  cfblk9/1 -> cfblk17/1
  cfblk17/1 -> cfblk15/1(cfblk1)
  cfblk8/1 -> cfblk18/1
  cfblk18/1 -> cfblk12/3(cfblk11)
  cfblk19/1 -> cfblk12/4(cfblk12)
  cfblk5/1 -> cfblk20/1
  cfblk20/1 -> cfblk15/2(cfblk9)

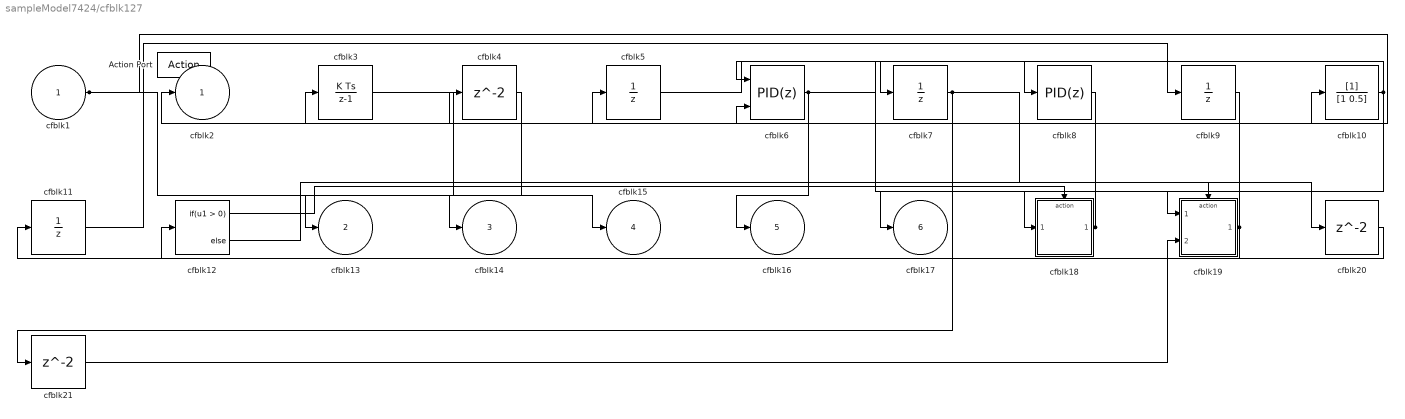
== system sampleModel7424/cfblk127 ==
  cfblk1 : Inport
  Action Port : ActionPort  ActionType=then
  cfblk10 : DiscreteFilter
  cfblk{5,7,9,11} (4 alike) : UnitDelay  SampleTime=-1
  cfblk12 : If  SampleTime=1
  cfblk18 : Subsystem  TreatAsAtomicUnit=on
  cfblk19 : Subsystem  TreatAsAtomicUnit=on
  cfblk20 : Delay
  cfblk21 : Delay
  cfblk3 : DiscreteIntegrator  InitialConditionSetting=State (most efficient)  SampleTime=-1  ICPrevOutput=DiscIntNeverNeededParam  ICPrevScaledInput=DiscIntNeverNeededParam
  cfblk4 : Delay
  cfblk6 : simulink/Continuous/PID Controller (2DOF)  Controller=PID  TimeDomain=Discrete-time  SampleTime=-1  IntegratorMethod=Forward Euler  FilterMethod=Forward Euler  Form=Parallel  UseFilter=on  ControllerParametersSource=internal  P=1  I=1  D=0  N=100  b=1  c=1  InitialConditionSource=internal  InitialConditionForIntegrator=0  InitialConditionForFilter=0  ExternalReset=none  LimitOutput=off  UpperSaturationLimit=inf  LowerSaturationLimit=-inf  LinearizeAsGain=off  AntiWindupMode=none  Kb=1  TrackingMode=off  Kt=1  PParamMin=[]  PParamMax=[]  IParamMin=[]  IParamMax=[]  DParamMin=[]  DParamMax=[]  NParamMin=[]  NParamMax=[]  bParamMin=[]  bParamMax=[]  cParamMin=[]  cParamMax=[]  KbParamMin=[]  KbParamMax=[]  KtParamMin=[]  KtParamMax=[]  POutMin=[]  POutMax=[]  IOutMin=[]  IOutMax=[]  DOutMin=[]  DOutMax=[]  NOutMin=[]  NOutMax=[]  bOutMin=[]  bOutMax=[]  cOutMin=[]  cOutMax=[]  KbOutMin=[]  KbOutMax=[]  KtOutMin=[]  KtOutMax=[]  IntegratorOutMin=[]  IntegratorOutMax=[]  FilterOutMin=[]  FilterOutMax=[]  SumOutMin=[]  SumOutMax=[]  Sum1OutMin=[]  Sum1OutMax=[]  Sum2OutMin=[]  Sum2OutMax=[]  Sum3OutMin=[]  Sum3OutMax=[]  SumI1OutMin=[]  SumI1OutMax=[]  SumI2OutMin=[]  SumI2OutMax=[]  SumI3OutMin=[]  SumI3OutMax=[]  SumDOutMin=[]  SumDOutMax=[]  SaturationOutMin=[]  SaturationOutMax=[]  IntegratorContinuousStateAttributes=''  IntegratorStateMustResolveToSignalObject=off  IntegratorRTWStateStorageClass=Auto  FilterContinuousStateAttributes=''  FilterStateMustResolveToSignalObject=off  FilterRTWStateStorageClass=Auto  DifferentiatorICPrevScaledInput=0  DifferentiatorOutMin=[]  DifferentiatorOutMax=[]  InitialConditionSetting=State (most efficient)
  cfblk8 : simulink/Continuous/PID Controller  Controller=PID  TimeDomain=Discrete-time  SampleTime=-1  IntegratorMethod=Forward Euler  FilterMethod=Forward Euler  Form=Parallel  UseFilter=on  ControllerParametersSource=internal  P=1  I=1  D=0  N=100  InitialConditionSource=internal  InitialConditionForIntegrator=0  InitialConditionForFilter=0  ExternalReset=none  LimitOutput=off  UpperSaturationLimit=inf  LowerSaturationLimit=-inf  LinearizeAsGain=off  AntiWindupMode=none  Kb=1  TrackingMode=off  Kt=1  PParamMin=[]  PParamMax=[]  IParamMin=[]  IParamMax=[]  DParamMin=[]  DParamMax=[]  NParamMin=[]  NParamMax=[]  KbParamMin=[]  KbParamMax=[]  KtParamMin=[]  KtParamMax=[]  POutMin=[]  POutMax=[]  IOutMin=[]  IOutMax=[]  DOutMin=[]  DOutMax=[]  NOutMin=[]  NOutMax=[]  KbOutMin=[]  KbOutMax=[]  KtOutMin=[]  KtOutMax=[]  IntegratorOutMin=[]  IntegratorOutMax=[]  FilterOutMin=[]  FilterOutMax=[]  SumOutMin=[]  SumOutMax=[]  SumI1OutMin=[]  SumI1OutMax=[]  SumI2OutMin=[]  SumI2OutMax=[]  SumI3OutMin=[]  SumI3OutMax=[]  SumDOutMin=[]  SumDOutMax=[]  SaturationOutMin=[]  SaturationOutMax=[]  IntegratorContinuousStateAttributes=''  IntegratorStateMustResolveToSignalObject=off  IntegratorRTWStateStorageClass=Auto  FilterContinuousStateAttributes=''  FilterStateMustResolveToSignalObject=off  FilterRTWStateStorageClass=Auto  DifferentiatorICPrevScaledInput=0  DifferentiatorOutMin=[]  DifferentiatorOutMax=[]  InitialConditionSetting=State (most efficient)
  cfblk2 : Outport
  cfblk13 : Outport  Port=2
  cfblk14 : Outport  Port=3
  cfblk15 : Outport  Port=4
  cfblk16 : Outport  Port=5
  cfblk17 : Outport  Port=6
  wires:
  cfblk9/1 -> cfblk17/1
  cfblk8/1 -> cfblk2/1
  cfblk7/1 -> cfblk20/1, cfblk21/1
  cfblk19/1(cfblk2) -> cfblk5/1, cfblk11/1
  cfblk11/1 -> cfblk9/1
  cfblk5/1 -> cfblk7/1
  cfblk18/1(cfblk2) -> cfblk3/1, cfblk4/1
  cfblk10/1 -> cfblk6/1, cfblk6/2, cfblk18/1(cfblk1)
  cfblk6/1 -> cfblk8/1, cfblk19/1(cfblk1), cfblk16/1
  cfblk4/1 -> cfblk13/1
  cfblk1/1 -> cfblk10/1, cfblk14/1
  cfblk3/1 -> cfblk15/1
  cfblk12/1 -> cfblk18/Action
  cfblk12/2 -> cfblk19/Action
  cfblk20/1 -> cfblk12/1
  cfblk21/1 -> cfblk19/2(cfblk10)

== system sampleModel7424/cfblk128 ==
  cfblk1 : Inport
  cfblk9 : Inport  Port=2
  cfblk10 : Inport  Port=3
  Action Port : ActionPort  ActionType=else
  cfblk13 : DataTypeConversion
  cfblk14 : DataTypeConversion
  cfblk3 : simulink/Discrete/Transfer Fcn Lead or Lag  PoleZ=0.95  ZeroZ=0.75  ICPrevOutput=0.0  ICPrevInput=0.0  DoSatur=off
      settings: SourceProductName=Simulink  SourceProductBaseCode=SL
  cfblk4 : DiscreteIntegrator  InitialConditionSetting=State (most efficient)  SampleTime=-1  ICPrevOutput=DiscIntNeverNeededParam  ICPrevScaledInput=DiscIntNeverNeededParam
  cfblk5 : UnitDelay  SampleTime=-1
  cfblk6 : simulink/Discrete/Transfer Fcn First Order  PoleZ=0.95  ICPrevOutput=0.0  DoSatur=off
      settings: SourceProductName=Simulink
  cfblk7 : DiscreteStateSpace  SampleTime=-1
  cfblk8 : simulink/Discrete/Transfer Fcn Real Zero  ZeroZ=0.75  ICPrevInput=0.0  DoSatur=off
      settings: SourceProductName=Simulink  SourceProductBaseCode=SL
  cfblk2 : Outport
  cfblk11 : Outport  Port=2
  cfblk12 : Outport  Port=3
  wires:
  cfblk9/1 -> cfblk5/1
  cfblk3/1 -> cfblk8/1
  cfblk5/1 -> cfblk11/1
  cfblk7/1 -> cfblk12/1
  cfblk10/1 -> cfblk2/1
  cfblk1/1 -> cfblk3/1
  cfblk8/1 -> cfblk6/1
  cfblk4/1 -> cfblk13/1
  cfblk13/1 -> cfblk7/1
  cfblk6/1 -> cfblk14/1
  cfblk14/1 -> cfblk4/1

== system sampleModel7424/cfblk129 ==
  cfblk1 : Inport
  cfblk8 : Inport  Port=2
  Action Port : ActionPort  ActionType=then
  cfblk10 : Delay
  cfblk3 : UnitDelay  SampleTime=-1
  cfblk4 : simulink/Continuous/PID Controller (2DOF)  Controller=PID  TimeDomain=Discrete-time  SampleTime=-1  IntegratorMethod=Forward Euler  FilterMethod=Forward Euler  Form=Parallel  UseFilter=on  ControllerParametersSource=internal  P=1  I=1  D=0  N=100  b=1  c=1  InitialConditionSource=internal  InitialConditionForIntegrator=0  InitialConditionForFilter=0  ExternalReset=none  LimitOutput=off  UpperSaturationLimit=inf  LowerSaturationLimit=-inf  LinearizeAsGain=off  AntiWindupMode=none  Kb=1  TrackingMode=off  Kt=1  PParamMin=[]  PParamMax=[]  IParamMin=[]  IParamMax=[]  DParamMin=[]  DParamMax=[]  NParamMin=[]  NParamMax=[]  bParamMin=[]  bParamMax=[]  cParamMin=[]  cParamMax=[]  KbParamMin=[]  KbParamMax=[]  KtParamMin=[]  KtParamMax=[]  POutMin=[]  POutMax=[]  IOutMin=[]  IOutMax=[]  DOutMin=[]  DOutMax=[]  NOutMin=[]  NOutMax=[]  bOutMin=[]  bOutMax=[]  cOutMin=[]  cOutMax=[]  KbOutMin=[]  KbOutMax=[]  KtOutMin=[]  KtOutMax=[]  IntegratorOutMin=[]  IntegratorOutMax=[]  FilterOutMin=[]  FilterOutMax=[]  SumOutMin=[]  SumOutMax=[]  Sum1OutMin=[]  Sum1OutMax=[]  Sum2OutMin=[]  Sum2OutMax=[]  Sum3OutMin=[]  Sum3OutMax=[]  SumI1OutMin=[]  SumI1OutMax=[]  SumI2OutMin=[]  SumI2OutMax=[]  SumI3OutMin=[]  SumI3OutMax=[]  SumDOutMin=[]  SumDOutMax=[]  SaturationOutMin=[]  SaturationOutMax=[]  IntegratorContinuousStateAttributes=''  IntegratorStateMustResolveToSignalObject=off  IntegratorRTWStateStorageClass=Auto  FilterContinuousStateAttributes=''  FilterStateMustResolveToSignalObject=off  FilterRTWStateStorageClass=Auto  DifferentiatorICPrevScaledInput=0  DifferentiatorOutMin=[]  DifferentiatorOutMax=[]  InitialConditionSetting=State (most efficient)
  cfblk5 : simulink/Continuous/PID Controller (2DOF)  Controller=PID  TimeDomain=Discrete-time  SampleTime=-1  IntegratorMethod=Forward Euler  FilterMethod=Forward Euler  Form=Parallel  UseFilter=on  ControllerParametersSource=internal  P=1  I=1  D=0  N=100  b=1  c=1  InitialConditionSource=internal  InitialConditionForIntegrator=0  InitialConditionForFilter=0  ExternalReset=none  LimitOutput=off  UpperSaturationLimit=inf  LowerSaturationLimit=-inf  LinearizeAsGain=off  AntiWindupMode=none  Kb=1  TrackingMode=off  Kt=1  PParamMin=[]  PParamMax=[]  IParamMin=[]  IParamMax=[]  DParamMin=[]  DParamMax=[]  NParamMin=[]  NParamMax=[]  bParamMin=[]  bParamMax=[]  cParamMin=[]  cParamMax=[]  KbParamMin=[]  KbParamMax=[]  KtParamMin=[]  KtParamMax=[]  POutMin=[]  POutMax=[]  IOutMin=[]  IOutMax=[]  DOutMin=[]  DOutMax=[]  NOutMin=[]  NOutMax=[]  bOutMin=[]  bOutMax=[]  cOutMin=[]  cOutMax=[]  KbOutMin=[]  KbOutMax=[]  KtOutMin=[]  KtOutMax=[]  IntegratorOutMin=[]  IntegratorOutMax=[]  FilterOutMin=[]  FilterOutMax=[]  SumOutMin=[]  SumOutMax=[]  Sum1OutMin=[]  Sum1OutMax=[]  Sum2OutMin=[]  Sum2OutMax=[]  Sum3OutMin=[]  Sum3OutMax=[]  SumI1OutMin=[]  SumI1OutMax=[]  SumI2OutMin=[]  SumI2OutMax=[]  SumI3OutMin=[]  SumI3OutMax=[]  SumDOutMin=[]  SumDOutMax=[]  SaturationOutMin=[]  SaturationOutMax=[]  IntegratorContinuousStateAttributes=''  IntegratorStateMustResolveToSignalObject=off  IntegratorRTWStateStorageClass=Auto  FilterContinuousStateAttributes=''  FilterStateMustResolveToSignalObject=off  FilterRTWStateStorageClass=Auto  DifferentiatorICPrevScaledInput=0  DifferentiatorOutMin=[]  DifferentiatorOutMax=[]  InitialConditionSetting=State (most efficient)
  cfblk6 : UnitDelay  SampleTime=-1
  cfblk7 : simulink/Discrete/Transfer Fcn Lead or Lag  PoleZ=0.95  ZeroZ=0.75  ICPrevOutput=0.0  ICPrevInput=0.0  DoSatur=off
      settings: SourceProductName=Simulink  SourceProductBaseCode=SL
  cfblk2 : Outport
  cfblk9 : Outport  Port=2
  wires:
  cfblk7/1 -> cfblk9/1
  cfblk8/1 -> cfblk2/1, cfblk5/2, cfblk3/1
  cfblk1/1 -> cfblk7/1
  cfblk3/1 -> cfblk4/1
  cfblk4/1 -> cfblk6/1
  cfblk6/1 -> cfblk5/1
  cfblk5/1 -> cfblk10/1
  cfblk10/1 -> cfblk4/2

== system sampleModel7424/cfblk130 ==
  cfblk1 : Inport
  cfblk7 : Inport  Port=2
  cfblk8 : Inport  Port=3
  Action Port : ActionPort  ActionType=else
  cfblk11 : Subsystem  TreatAsAtomicUnit=on
  cfblk12 : Subsystem  TreatAsAtomicUnit=on
  cfblk13 : Delay
  cfblk14 : Delay
  cfblk3 : DiscreteFir
  cfblk4 : simulink/Continuous/PID Controller  Controller=PID  TimeDomain=Discrete-time  SampleTime=-1  IntegratorMethod=Forward Euler  FilterMethod=Forward Euler  Form=Parallel  UseFilter=on  ControllerParametersSource=internal  P=1  I=1  D=0  N=100  InitialConditionSource=internal  InitialConditionForIntegrator=0  InitialConditionForFilter=0  ExternalReset=none  LimitOutput=off  UpperSaturationLimit=inf  LowerSaturationLimit=-inf  LinearizeAsGain=off  AntiWindupMode=none  Kb=1  TrackingMode=off  Kt=1  PParamMin=[]  PParamMax=[]  IParamMin=[]  IParamMax=[]  DParamMin=[]  DParamMax=[]  NParamMin=[]  NParamMax=[]  KbParamMin=[]  KbParamMax=[]  KtParamMin=[]  KtParamMax=[]  POutMin=[]  POutMax=[]  IOutMin=[]  IOutMax=[]  DOutMin=[]  DOutMax=[]  NOutMin=[]  NOutMax=[]  KbOutMin=[]  KbOutMax=[]  KtOutMin=[]  KtOutMax=[]  IntegratorOutMin=[]  IntegratorOutMax=[]  FilterOutMin=[]  FilterOutMax=[]  SumOutMin=[]  SumOutMax=[]  SumI1OutMin=[]  SumI1OutMax=[]  SumI2OutMin=[]  SumI2OutMax=[]  SumI3OutMin=[]  SumI3OutMax=[]  SumDOutMin=[]  SumDOutMax=[]  SaturationOutMin=[]  SaturationOutMax=[]  IntegratorContinuousStateAttributes=''  IntegratorStateMustResolveToSignalObject=off  IntegratorRTWStateStorageClass=Auto  FilterContinuousStateAttributes=''  FilterStateMustResolveToSignalObject=off  FilterRTWStateStorageClass=Auto  DifferentiatorICPrevScaledInput=0  DifferentiatorOutMin=[]  DifferentiatorOutMax=[]  InitialConditionSetting=State (most efficient)
  cfblk5 : UnitDelay  SampleTime=-1
  cfblk6 : If  SampleTime=1
  cfblk2 : Outport
  cfblk9 : Outport  Port=2
  cfblk10 : Outport  Port=3
  wires:
  cfblk11/1(cfblk2) -> cfblk3/1
  cfblk7/1 -> cfblk4/1
  cfblk1/1 -> cfblk11/1(cfblk1), cfblk12/3(cfblk14)
  cfblk11/2(cfblk10) -> cfblk2/1
  cfblk11/3(cfblk11) -> cfblk9/1, cfblk12/4(cfblk15)
  cfblk8/1 -> cfblk6/1, cfblk12/5(cfblk16)
  cfblk3/1 -> cfblk5/1
  cfblk4/1 -> cfblk12/2(cfblk13)
  cfblk12/1(cfblk2) -> cfblk10/1
  cfblk6/1 -> cfblk11/Action
  cfblk6/2 -> cfblk12/Action
  cfblk5/1 -> cfblk13/1
  cfblk13/1 -> cfblk12/1(cfblk1)
  cfblk12/2(cfblk17) -> cfblk14/1
  cfblk14/1 -> cfblk11/2(cfblk9)

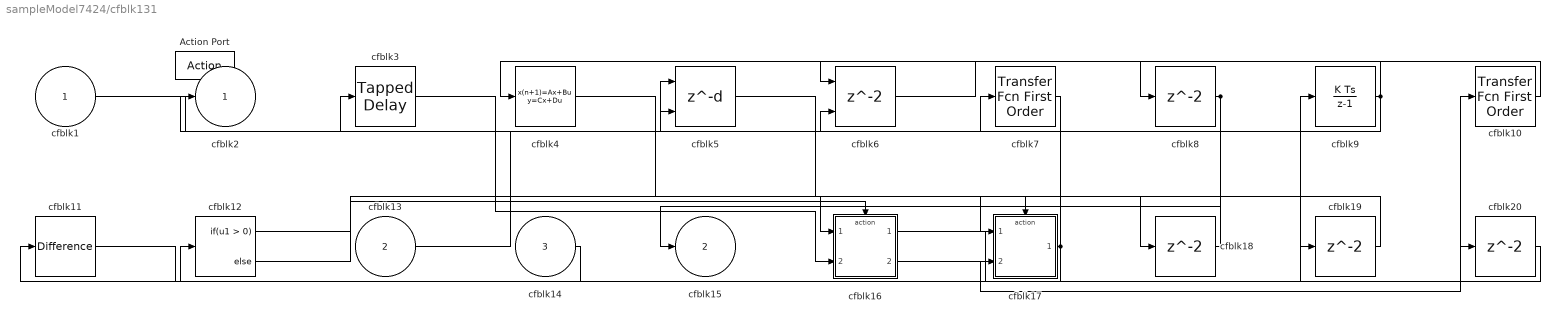
== system sampleModel7424/cfblk131 ==
  cfblk1 : Inport
  cfblk13 : Inport  Port=2
  cfblk14 : Inport  Port=3
  Action Port : ActionPort  ActionType=then
  cfblk10 : simulink/Discrete/Transfer Fcn First Order  PoleZ=0.95  ICPrevOutput=0.0  DoSatur=off
      settings: SourceProductName=Simulink
  cfblk11 : simulink/Discrete/Difference  ICPrevInput=0.0  OutMin=[]  OutMax=[]  OutDataTypeStr=Inherit: Inherit via back propagation  OutDataType=fixdt(1, 16)  OutScaling=2^-10  DoSatur=off
  cfblk12 : If  SampleTime=1
  cfblk16 : Subsystem  TreatAsAtomicUnit=on
  cfblk17 : Subsystem  TreatAsAtomicUnit=on
  cfblk{8,18..20} (4 alike) : Delay
  cfblk3 : simulink/Discrete/Tapped Delay  vinit=0.0  samptime=-1  NumDelays=1  DelayOrder=Oldest  includeCurrent=off
  cfblk4 : DiscreteStateSpace  SampleTime=-1
  cfblk5 : Delay  DelayLengthSource=Input port
      settings: InputPortMap=u0,p1
  cfblk6 : Delay  ShowEnablePort=on
      settings: InputPortMap=u0,e6
  cfblk7 : simulink/Discrete/Transfer Fcn First Order  PoleZ=0.95  ICPrevOutput=0.0  DoSatur=off
      settings: SourceProductName=Simulink
  cfblk9 : DiscreteIntegrator  InitialConditionSetting=State (most efficient)  SampleTime=-1  ICPrevOutput=DiscIntNeverNeededParam  ICPrevScaledInput=DiscIntNeverNeededParam
  cfblk2 : Outport
  cfblk15 : Outport  Port=2
  wires:
  cfblk10/1 -> cfblk4/1
  cfblk13/1 -> cfblk7/1
  cfblk9/1 -> cfblk6/1, cfblk2/1
  cfblk1/1 -> cfblk3/1
  cfblk17/1(cfblk2) -> cfblk5/1, cfblk11/1
  cfblk6/1 -> cfblk8/1
  cfblk16/1(cfblk2) -> cfblk9/1
  cfblk16/2(cfblk13) -> cfblk10/1
  cfblk14/1 -> cfblk12/1
  cfblk3/1 -> cfblk16/2(cfblk12)
  cfblk7/1 -> cfblk6/2
  cfblk8/1 -> cfblk5/2, cfblk15/1
  cfblk12/1 -> cfblk16/Action
  cfblk12/2 -> cfblk17/Action
  cfblk5/1 -> cfblk18/1
  cfblk18/1 -> cfblk16/1(cfblk1)
  cfblk4/1 -> cfblk19/1
  cfblk19/1 -> cfblk17/1(cfblk1)
  cfblk11/1 -> cfblk20/1
  cfblk20/1 -> cfblk17/2(cfblk8)

== system sampleModel7424/cfblk132 ==
  cfblk1 : Inport
  cfblk13 : Inport  Port=2
  cfblk14 : Inport  Port=3
  Action Port : ActionPort  ActionType=else
  cfblk10 : simulink/Continuous/PID Controller (2DOF)  Controller=PID  TimeDomain=Discrete-time  SampleTime=-1  IntegratorMethod=Forward Euler  FilterMethod=Forward Euler  Form=Parallel  UseFilter=on  ControllerParametersSource=internal  P=1  I=1  D=0  N=100  b=1  c=1  InitialConditionSource=internal  InitialConditionForIntegrator=0  InitialConditionForFilter=0  ExternalReset=none  LimitOutput=off  UpperSaturationLimit=inf  LowerSaturationLimit=-inf  LinearizeAsGain=off  AntiWindupMode=none  Kb=1  TrackingMode=off  Kt=1  PParamMin=[]  PParamMax=[]  IParamMin=[]  IParamMax=[]  DParamMin=[]  DParamMax=[]  NParamMin=[]  NParamMax=[]  bParamMin=[]  bParamMax=[]  cParamMin=[]  cParamMax=[]  KbParamMin=[]  KbParamMax=[]  KtParamMin=[]  KtParamMax=[]  POutMin=[]  POutMax=[]  IOutMin=[]  IOutMax=[]  DOutMin=[]  DOutMax=[]  NOutMin=[]  NOutMax=[]  bOutMin=[]  bOutMax=[]  cOutMin=[]  cOutMax=[]  KbOutMin=[]  KbOutMax=[]  KtOutMin=[]  KtOutMax=[]  IntegratorOutMin=[]  IntegratorOutMax=[]  FilterOutMin=[]  FilterOutMax=[]  SumOutMin=[]  SumOutMax=[]  Sum1OutMin=[]  Sum1OutMax=[]  Sum2OutMin=[]  Sum2OutMax=[]  Sum3OutMin=[]  Sum3OutMax=[]  SumI1OutMin=[]  SumI1OutMax=[]  SumI2OutMin=[]  SumI2OutMax=[]  SumI3OutMin=[]  SumI3OutMax=[]  SumDOutMin=[]  SumDOutMax=[]  SaturationOutMin=[]  SaturationOutMax=[]  IntegratorContinuousStateAttributes=''  IntegratorStateMustResolveToSignalObject=off  IntegratorRTWStateStorageClass=Auto  FilterContinuousStateAttributes=''  FilterStateMustResolveToSignalObject=off  FilterRTWStateStorageClass=Auto  DifferentiatorICPrevScaledInput=0  DifferentiatorOutMin=[]  DifferentiatorOutMax=[]  InitialConditionSetting=State (most efficient)
  cfblk11 : Delay
  cfblk12 : DiscreteFilter
  cfblk15 : Delay
  cfblk3 : simulink/Discrete/Transfer Fcn Real Zero  ZeroZ=0.75  ICPrevInput=0.0  DoSatur=off
      settings: SourceProductName=Simulink  SourceProductBaseCode=SL
  cfblk4 : DiscreteFir
  cfblk5 : DiscreteFilter
  cfblk6 : DiscreteIntegrator  InitialConditionSetting=State (most efficient)  SampleTime=-1  ICPrevOutput=DiscIntNeverNeededParam  ICPrevScaledInput=DiscIntNeverNeededParam
  cfblk7 : Delay  ShowEnablePort=on
      settings: InputPortMap=u0,e6
  cfblk8 : Delay  DelayLengthSource=Input port
      settings: InputPortMap=u0,p1
  cfblk9 : simulink/Discrete/Transfer Fcn First Order  PoleZ=0.95  ICPrevOutput=0.0  DoSatur=off
      settings: SourceProductName=Simulink
  cfblk2 : Outport
  wires:
  cfblk8/1 -> cfblk7/1
  cfblk6/1 -> cfblk12/1
  cfblk4/1 -> cfblk10/1
  cfblk12/1 -> cfblk7/2
  cfblk7/1 -> cfblk3/1
  cfblk5/1 -> cfblk10/2
  cfblk14/1 -> cfblk11/1
  cfblk13/1 -> cfblk4/1, cfblk9/1
  cfblk10/1 -> cfblk8/2
  cfblk1/1 -> cfblk5/1
  cfblk11/1 -> cfblk2/1
  cfblk9/1 -> cfblk6/1
  cfblk3/1 -> cfblk15/1
  cfblk15/1 -> cfblk8/1
